simulink model "Chapter_9_Section_3_1"  (R2026a)
settings: Solver=FixedStepAuto  StopTime=500  FixedStep=0.02  EnableMultiTasking=on
libraries: arduinolib x1, simulink x1
settings Model: SimulationMode=external  SILPILModeSetting=veronly  ExtModeTrigDuration=2  Creator=ASUS  LastModifiedBy=ASUS
settings HardwareCC: ProdBitPerInt=16.0  ProdBitPerPointer=16.0  ProdBitPerSizeT=16.0  ProdBitPerPtrDiffT=16.0  ProdWordSize=8.0  ProdHWDeviceType=Atmel->AVR  UseEmbeddedCoderFeatures=off
settings RTWCC: SystemTargetFile=ert.tlc  HardwareBoard=Arduino Mega 2560  TLCOptions=-aInlineSetEventsForThisBaseRateFcn=TLC_FALSE -aSuppressMultiTaskScheduler=TLC_FALSE -aRateBasedStepFcn=1  Toolchain=Arduino AVR  BuildConfiguration=Specify  Description=Embedded Coder
settings ERTTargetCC: ExtModeTransport=3.0  ExtModeAutomaticAllocSize=off  ExtModeStaticAllocSize=2048.0  SupportContinuousTime=on  SupportNonInlinedSFcns=on  SupportVariableSizeSignals=on

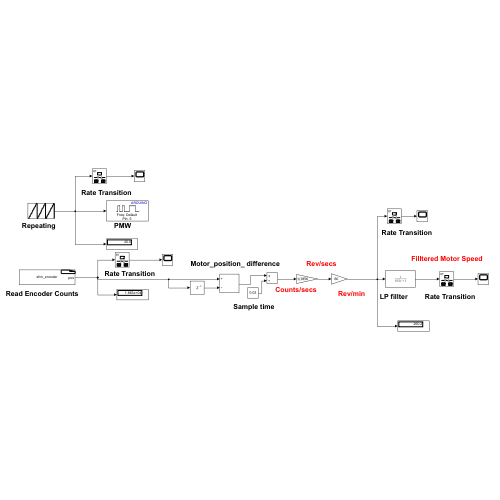
[thumbnail: Simulink's stored preview of the top-level diagram]
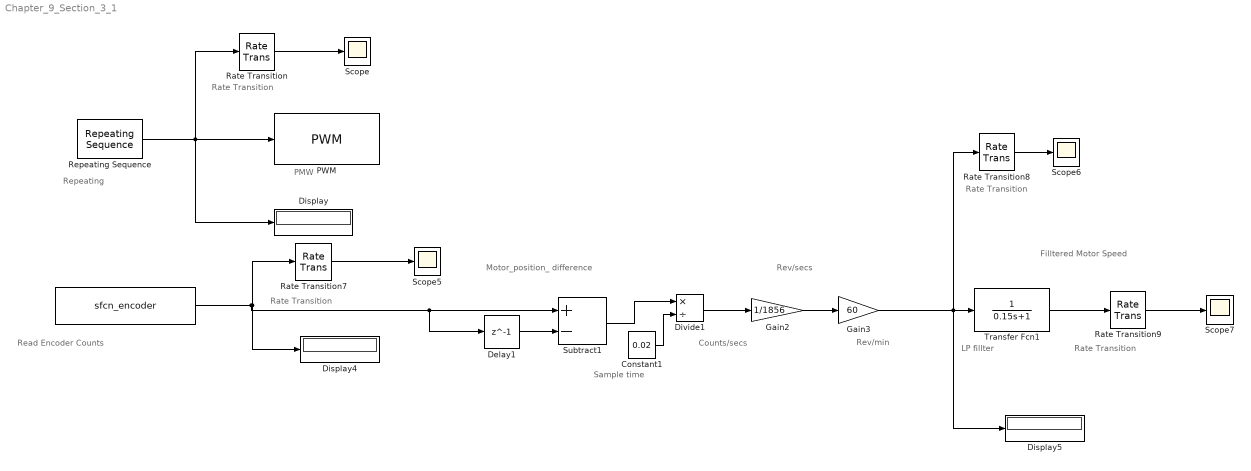
== system Chapter_9_Section_3_1 ==
  note: Rate Transition
  note: Repeating
  note: PMW
  note: Read Encoder Counts
  note: Rate Transition
  note: Rate Transition
  note: Rate Transition
  note: Sample time
  note: Motor_position_ difference
  note: Counts/secs
  note: Rev/secs
  note: Rev/min
  note: LP fillter
  note: Filltered Motor Speed
  " " : S-Function  InitFcn=try, set_param(gcb,'FunctionName','sfcn_encoder'), end  FunctionName=sfcn_encoder  Parameters=uint8(0),uint8(2),uint8(3)  SFunctionModules=sfcn_encoder_wrapper.c  SFunctionDeploymentMode=off  EnableBusSupport=off  mask(S-Function Builder){}
      mask init:
      | val = [[.9  0.75 0.75 1 1 .9 .9 1]',[1 1 0.75 0.75 .9 .9 1 .9]'];try , sys = get_param(gcb,'SfunBuilderFcnName');if isempty(sys), sys = get_param(gcb,'FunctionName'); end,catch, sys = get_param(gcb,'FunctionName'); end
      settings: CopyFcn=set_param(gcbh,'LinkStatus','none')  PreSaveFcn=try, set_param(gcb,'FunctionName','sfcn_encoder'), end  OpenFcn=sfunctionwizard(gcbh)
      mask Display:
      | plot(val(:,1),val(:,2))
      | disp(sys)
      | port_label('output',1,sprintf('%s', 'pos'),'interpreter','tex')
  Constant1 : Constant  Value=0.02
  Delay1 : Delay  DelayLength=1  InitialCondition=0
  Display : Display
  Display4 : Display
  Display5 : Display
  Divide1 : Product  Inputs=*/
  Gain2 : Gain  Gain=1/1856
  Gain3 : Gain  Gain=60
  PWM : arduinolib/PWM  pinNumber=5  frequencyType=Default  desiredFrequency=490.2  achievableFrequency=490.1961
  Rate Transition{,7..9} (4 alike) : RateTransition
  Repeating Sequence : simulink/Sources/Repeating Sequence  rep_seq_t=[0 49.9 50 99.9 100 149.9 150 199.9 200 249.9 250 299.9 300 349.9 350 399.9 400 449.9 450 500]  rep_seq_y=[25.5 25.5 50.1 50.1 76.5 76.5 102 102 127.5 127.5 153 153 178.5 178.5 204 204 229.5 229.5 255 255]
  Scope{,5..7} (4 alike) : Scope
      Scope settings: ActiveDisplayYMinimum=-214.23426486198696  ActiveDisplayYMaximum=571.66849156764079  DataLoggingVariableName=PWM_Input  DataLoggingSaveFormat=Array
      Scope5 settings: ActiveDisplayYMinimum=-22.407200582277603  ActiveDisplayYMaximum=19.171363005949797  DataLoggingVariableName=ScopeData5
      Scope6 settings: ActiveDisplayYMinimum=-397.50774034878805  ActiveDisplayYMaximum=278.06370212636983  DataLoggingVariableName=ScopeData6
      Scope7 settings: ActiveDisplayYMinimum=-145.40819031202872  ActiveDisplayYMaximum=451.42076984791106  DataLoggingVariableName=Motor_Speed_RPM_Filtered  DataLoggingSaveFormat=Array
  Subtract1 : Sum  Inputs=+-
  Transfer Fcn1 : TransferFcn  Denominator=[0.15 1]
  wires:
  " "/1 -> Display4/1, Rate Transition7/1, Delay1/1, Subtract1/1
  Rate Transition7/1 -> Scope5/1
  Repeating Sequence/1 -> Display/1, Rate Transition/1, PWM/1
  Rate Transition/1 -> Scope/1
  Gain2/1 -> Gain3/1
  Divide1/1 -> Gain2/1
  Rate Transition9/1 -> Scope7/1
  Rate Transition8/1 -> Scope6/1
  Constant1/1 -> Divide1/2
  Transfer Fcn1/1 -> Rate Transition9/1
  Delay1/1 -> Subtract1/2
  Subtract1/1 -> Divide1/1
  Gain3/1 -> Transfer Fcn1/1, Display5/1, Rate Transition8/1
